simulink model "model_nl_out"  (R2020b)
settings: Solver=FixedStepAuto  StartTime=t(1)  StopTime=t(end)  FixedStep=1/harm.fs  RelTol=1e-3
values from neighbouring files (symbols this model uses):
  even_nl_amp = 0.001    [Tutorial_3_nonlinear_in.m]    (also in Tutorial_3_nonlinear_out.m = 1)
  odd_nl_amp = 0.0001    [Tutorial_3_nonlinear_in.m]    (also in Tutorial_3_nonlinear_out.m = 0.1)
libraries: cstblocks x1
settings Model: Creator=ohnishi  LastModifiedBy=ohnishi

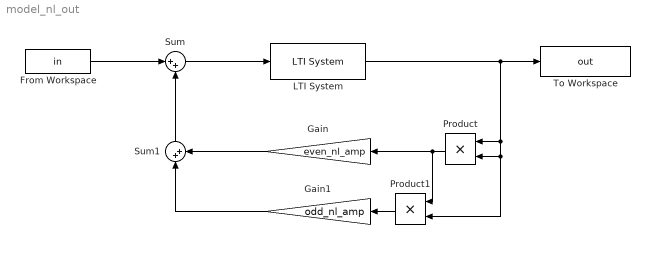
== system model_nl_out ==
  From Workspace : FromWorkspace  VariableName=in
  Gain : Gain  Gain=even_nl_amp
  Gain1 : Gain  Gain=odd_nl_amp
  LTI System : cstblocks/LTI System  sys=G  IC=[]
  Product : Product
  Product1 : Product
  Sum : Sum  Inputs=|++
  Sum1 : Sum  Inputs=|++
  To Workspace : ToWorkspace  VariableName=out  SampleTime=-1
  wires:
  From Workspace/1 -> Sum/1
  Sum/1 -> LTI System/1
  LTI System/1 -> Product1/2, Product/2, Product/1, To Workspace/1
  Product/1 -> Product1/1, Gain/1
  Product1/1 -> Gain1/1
  Gain/1 -> Sum1/2
  Gain1/1 -> Sum1/1
  Sum1/1 -> Sum/2
